simulink model "sl_puma_hw7"  (R2016a)
settings: Solver=ode45  StartTime=0.0  StopTime=10  FixedStep=.001  RelTol=1e-3
libraries: roblocks x2
settings Model: ExtModeTrigMode=oneshot  ExtModeArmWhenConnect=off  Creator=pic  LastModifiedBy=magiccjae
settings DataIOCC: SaveFormat=Array  SignalLoggingSaveFormat=ModelDataLogs  SignalLogging=off  ReturnWorkspaceOutputs=on
settings OptimizationCC: BlockReduction=off  BooleanDataType=off  ExpressionDepthLimit=2147483647  InitFltsAndDblsToZero=on
settings DebuggingCC: SaveWithParameterizedLinksMsg=none  UnderspecifiedInitializationDetection=Classic  MergeDetectMultiDrivingBlocksExec=none  SignalResolutionControl=TryResolveAllWithWarning  MultiTaskDSMMsg=warning  MultiTaskCondExecSysMsg=none  FcnCallInpInsideContextMsg=EnableAllAsWarning  StateNameClashWarn=warning
settings HardwareCC: ProdBitPerPointer=32  ProdLargestAtomicFloat=None  ProdIntDivRoundTo=Undefined  ProdEndianess=Unspecified  ProdWordSize=32  ProdHWDeviceType=32-bit Generic  TargetUnknown=on
settings ModelReferenceCC: PropagateSignalLabelsOutOfModel=off
settings GRTTargetCC: ModelReferenceCompliant=off  ParMdlRefBuildCompliant=off  CompOptLevelCompliant=off  CombineOutputUpdateFcns=off  MatFileLogging=off  GRTInterface=on
settings ConfigComp: CovModelRefEnable=Off  CovSFcnEnable=off

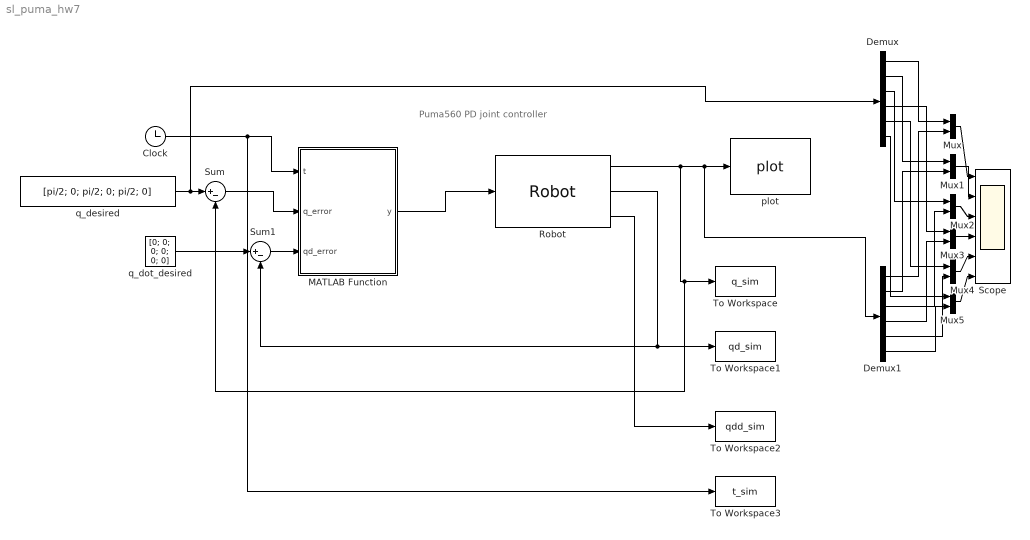
== system sl_puma_hw7 ==
  note: Puma560 PD joint controller
  Clock : Clock
  Demux : Demux  Outputs=6
  Demux1 : Demux  Outputs=6
  MATLAB Function : MATLAB Function  TreatAsAtomicUnit=on
  Mux{,1..5} (6 alike) : Mux  Inputs=2
  Robot : roblocks/Dynamics/Robot  robot=p560.nofriction  q0=[0 0 0 0 0 0]
  Scope : Scope  NumInputPorts=6
  Sum : Sum  Inputs=|+-
  Sum1 : Sum  Inputs=|+-
  To Workspace : ToWorkspace  VariableName=q_sim  SampleTime=-1
  To Workspace1 : ToWorkspace  VariableName=qd_sim  SampleTime=-1
  To Workspace2 : ToWorkspace  VariableName=qdd_sim  SampleTime=-1
  To Workspace3 : ToWorkspace  VariableName=t_sim  SampleTime=-1
  plot : roblocks/Robot Graphics/plot  robot=p560  fps=25  holdplot=on
  q_desired : Constant  Value=[pi/2; 0; pi/2; 0; pi/2; 0]
  q_dot_desired : Constant  Value=[0; 0; 0; 0; 0; 0]
  wires:
  Robot/1 -> Sum/2, To Workspace/1, Demux1/1, plot/1
  Robot/3 -> To Workspace2/1
  Robot/2 -> To Workspace1/1, Sum1/2
  MATLAB Function/1(y) -> Robot/1
  Clock/1 -> To Workspace3/1, MATLAB Function/1(t)
  q_desired/1 -> Demux/1, Sum/1
  q_dot_desired/1 -> Sum1/1
  Sum/1 -> MATLAB Function/2(q_error)
  Sum1/1 -> MATLAB Function/3(qd_error)
  Mux/1 -> Scope/1
  Demux/1 -> Mux/1
  Demux1/1 -> Mux/2
  Demux/2 -> Mux1/1
  Demux1/2 -> Mux1/2
  Mux1/1 -> Scope/2
  Mux2/1 -> Scope/3
  Demux/3 -> Mux2/1
  Demux1/3 -> Mux2/2
  Mux3/1 -> Scope/4
  Demux/4 -> Mux3/1
  Demux1/4 -> Mux3/2
  Mux4/1 -> Scope/5
  Demux/5 -> Mux4/1
  Demux1/5 -> Mux4/2
  Mux5/1 -> Scope/6
  Demux/6 -> Mux5/1
  Demux1/6 -> Mux5/2

== matlab function sl_puma_hw7/MATLAB Function ==
  data: t input; y output; q_error input; qd_error input
function y = get_torque(t, q_error, qd_error)


Kp = [10 0 0 0 0 0;...
      0 1000 0 0 0 0;...
      0 0 1000 0 0 0;...
      0 0 0 10 0 0;...
      0 0 0 0 10 0;...
      0 0 0 0 0 10];

Kd = [1 0 0 0 0 0;...
      0 100 0 0 0 0;...
      0 0 100 0 0 0;...
      0 0 0 1 0 0;...
      0 0 0 0 1 0;...
      0 0 0 0 0 1];
  
y = Kp*q_error + Kd*qd_error;

end
